simulink model "inverter"  (R2020b)
settings: Solver=VariableStepAuto  StartTime=0.0  StopTime=0.1  MaxStep=1e-7  MinStep=1e-8  RelTol=1e-3
libraries: powerlib x14, simulink x1
settings Model: Creator=dhill12g  LastModifiedBy=asfourm

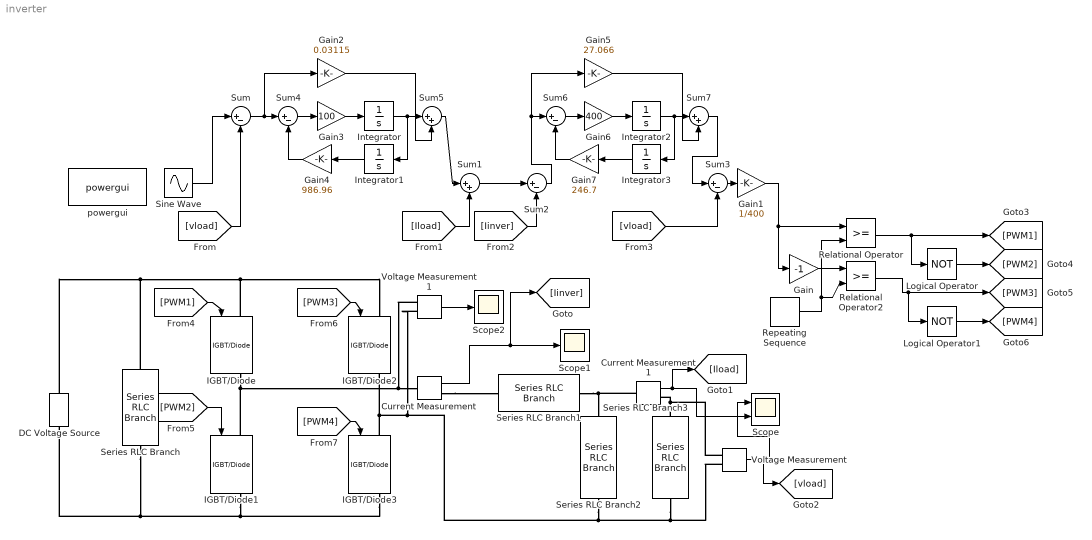
== system inverter ==
  Current Measurement : powerlib/Measurements/Current Measurement  PhasorSimulation=off  OutputType=Complex  PSBequivalent=0
  Current Measurement1 : powerlib/Measurements/Current Measurement  PhasorSimulation=off  OutputType=Complex  PSBequivalent=0
  DC Voltage Source : powerlib/Electrical Sources/DC Voltage Source  Amplitude=380  Measurements=None
  Gain : Gain  Gain=-1
  Gain1 : Gain  Gain=1/400
  Gain2 : Gain  Gain=0.03115
  Gain3 : Gain  Gain=100
  Gain4 : Gain  Gain=986.96
  Gain5 : Gain  Gain=27.066
  Gain6 : Gain  Gain=400
  Gain7 : Gain  Gain=246.7
  IGBT/Diode{,1..3} (4 alike) : powerlib/Power Electronics/IGBT//Diode  Ron=1e-3  Rs=1e5  Cs=inf  Measurements=on
  Integrator{,1..3} (4 alike) : Integrator
  Logical Operator : Logic  Operator=NOT  AllPortsSameDT=off  OutDataTypeStr=boolean
  Logical Operator1 : Logic  Operator=NOT  AllPortsSameDT=off  OutDataTypeStr=boolean
  Relational Operator : RelationalOperator  OutDataTypeStr=boolean  RndMeth=Simplest
  Relational Operator2 : RelationalOperator  OutDataTypeStr=boolean  RndMeth=Simplest
  Repeating Sequence : simulink/Sources/Repeating Sequence  rep_seq_t=[0 0.00005 0.0001]  rep_seq_y=[-1 1 -1]
  Scope : Scope  NumInputPorts=2
  Scope1 : Scope
  Scope2 : Scope
  Series RLC Branch : powerlib/Elements/Series RLC Branch  LConnTagsString=__new0  RConnTagsString=__new0  BranchType=RC  Resistance=0.0042  Inductance=1e-3  SetiL0=off  InitialCurrent=0  Capacitance=500e-6  Setx0=off  InitialVoltage=0  Measurements=None
  Series RLC Branch1 : powerlib/Elements/Series RLC Branch  LConnTagsString=__new0  RConnTagsString=__new0  BranchType=RL  Resistance=0.001  Inductance=4.06e-3  SetiL0=off  InitialCurrent=0  Capacitance=500e-6  Setx0=off  InitialVoltage=0  Measurements=None
  Series RLC Branch2 : powerlib/Elements/Series RLC Branch  LConnTagsString=__new0  RConnTagsString=__new0  BranchType=RC  Resistance=4e-3  Inductance=4.42e-3  SetiL0=off  InitialCurrent=0  Capacitance=6.23e-6  Setx0=off  InitialVoltage=0  Measurements=None
  Series RLC Branch3 : powerlib/Elements/Series RLC Branch  LConnTagsString=__new0  RConnTagsString=__new0  BranchType=R  Resistance=55  Inductance=4.42e-3  SetiL0=off  InitialCurrent=0  Capacitance=5.7e-6  Setx0=off  InitialVoltage=0  Measurements=None
  Sine Wave : Sin  Amplitude=120*sqrt(2)  Frequency=2*pi*50  SampleTime=0
  Sum{,2..4,6} (5 alike) : Sum  Inputs=|+-
  Sum1 : Sum  Inputs=|++
  Sum5 : Sum  Inputs=|++
  Sum7 : Sum  Inputs=|++
  Voltage Measurement : powerlib/Measurements/Voltage Measurement  PhasorSimulation=off  OutputType=Complex  PSBequivalent=0
  Voltage Measurement1 : powerlib/Measurements/Voltage Measurement  PhasorSimulation=off  OutputType=Complex  PSBequivalent=0
  powergui : powerlib/powergui  Priority=1  SimulationMode=Continuous  SampleTime=1e-06  frequency=60  Iterations=50  frequencyindice=0  Pbase=100e6  ErrMax=1e-4  UnitsV=kV  UnitsW=MW  buscounter=0  FunctionMessages=off  echomessages=off  EnableUseOfTLC=off  CurrentSourceSwitches=off  DisableSnubberDevices=off  DisableRonSwitches=off  DisableVfSwitches=off  DisplayEquations=off  AutomaticDiscreteSolvers=off  SolverType=Tustin/Backward Euler (TBE)  Interpol=off  ExternalGateDelay=off  methode=off  Ts=100  x0status=blocks  SPID=on  SwTol=0  HookPort=off  NonlinearTolerance=1e-4  nMaxIteration=100  ContinueOnMaxIteration=off  RestoreLinks=warning  ResistiveCurrentMeasurement=off  Frange=[0:2:500]  Ylog=off  Xlog=on  ShowGrid=off  save=off  variable=ZData  structure=0  ZoomFFT=off  StartTime=0.0  cycles=1  DisplayStyle=1  fundamental=60  FreqAxis=off  MaxFrequency=1000  frequencyindicesteady=1  RmsSteady=1  display=off
  wires:
  Current Measurement1/1 -> Scope/2, [Iload]
  Voltage Measurement/1 -> Scope/1, [vload]
  Current Measurement/1 -> [Iinver], Scope1/1
  Sine Wave/1 -> Sum/1
  [vload] -> Sum/2
  Sum/1 -> Gain2/1, Sum4/1
  [Iload] -> Sum1/2
  Sum1/1 -> Sum2/1
  [Iinver] -> Sum2/2
  Sum7/1 -> Sum3/1
  [vload] -> Sum3/2
  Sum3/1 -> Gain1/1
  Gain/1 -> Relational Operator2/1
  Repeating Sequence/1 -> Relational Operator/2, Relational Operator2/2
  Relational Operator/1 -> Logical Operator/1, [PWM1]
  Logical Operator/1 -> [PWM2]
  Logical Operator1/1 -> [PWM4]
  Relational Operator2/1 -> Logical Operator1/1, [PWM3]
  [PWM1] -> IGBT/Diode/1
  [PWM2] -> IGBT/Diode1/1
  [PWM3] -> IGBT/Diode2/1
  [PWM4] -> IGBT/Diode3/1
  Voltage Measurement1/1 -> Scope2/1
  Gain1/1 -> Gain/1, Relational Operator/1
  Sum4/1 -> Gain3/1
  Gain3/1 -> Integrator/1
  Gain4/1 -> Sum4/2
  Integrator1/1 -> Gain4/1
  Integrator/1 -> Sum5/1, Integrator1/1
  Sum5/1 -> Sum1/1
  Gain2/1 -> Sum5/2
  Sum2/1 -> Gain5/1, Sum6/1
  Gain5/1 -> Sum7/2
  Sum6/1 -> Gain6/1
  Gain6/1 -> Integrator2/1
  Integrator2/1 -> Sum7/1, Integrator3/1
  Gain7/1 -> Sum6/2
  Integrator3/1 -> Gain7/1
  connections:
  IGBT/Diode1/LConn1 -- Voltage Measurement1/LConn1 -- Current Measurement/LConn1 -- IGBT/Diode/RConn1
  IGBT/Diode3/LConn1 -- Voltage Measurement1/LConn2 -- Voltage Measurement/LConn2 -- Series RLC Branch3/RConn1 -- Series RLC Branch2/RConn1 -- IGBT/Diode2/RConn1
  IGBT/Diode3/RConn1 -- IGBT/Diode1/RConn1 -- DC Voltage Source/LConn1 -- Series RLC Branch/RConn1
  DC Voltage Source/RConn1 -- Series RLC Branch/LConn1 -- IGBT/Diode/LConn1 -- IGBT/Diode2/LConn1
  Current Measurement/RConn1 -- Series RLC Branch1/LConn1
  Series RLC Branch1/RConn1 -- Current Measurement1/LConn1 -- Series RLC Branch2/LConn1
  Series RLC Branch3/LConn1 -- Voltage Measurement/LConn1 -- Current Measurement1/RConn1
